simulink model "detumbling"  (R2020a)
settings: Solver=VariableStepAuto  StartTime=0.0  StopTime=3000  RelTol=1e-3
values from neighbouring files (symbols this model uses):
  a = (6371+h)*1e3    (= 6871000)    [AMM_main.m]    (also in Data.m)
  A_RW = sqrt([prop1;prop2;prop3]/(prop1+prop2+prop3))    [AMM_main.m]    (also in Data.m)
  A_t = [Ax;Ay;Az;Ax;Ay;Az;A_sp;A_sp;A_sp;A_sp;]    [AMM_main.m]    (also in Data.m)
  alpha = 0.005    [AMM_main.m]    (also in Data.m = 0.5)
  cd = 2.2    [AMM_main.m]    (also in Data.m)
  init_DCM = DCM0_track    [AMM_main.m]    (also in Data.m = [0.097540404999410   0.957506835434298   0.970592781760616)
  init_orb = orb0_track    [AMM_main.m]    (also in Data.m = [e0,i0,O0,o0,th0])
  init_tumbl = w0_track    [AMM_main.m]    (also in Data.m = 10*pi/180*dir)
  Ir = 1e-7    (= 1e-07)    [AMM_main.m]    (also in Data.m)
  Iz = 2e-7    (= 2e-07)    [AMM_main.m]    (also in Data.m)
  J = [Jx;Jy;Jz]    [AMM_main.m]    (also in Data.m)
  k_mt = 1e10    (= 10000000000)    [AMM_main.m]    (also in Data.m = 1000000)
  k_RW = .1    (= 0.1)    [AMM_main.m]    (also in Data.m = 1)
  max_mx = 1.19    [AMM_main.m]    (also in Data.m)
  max_my = 1.19    [AMM_main.m]    (also in Data.m)
  max_mz = 1.19    [AMM_main.m]    (also in Data.m)
  n = sqrt( mu / a^3 )    [AMM_main.m]    (also in Data.m)
  rho = [rho_sMB;rho_dMB;rho_sSP;rho_dSP]    [AMM_main.m]    (also in Data.m)
  rho_air = 4.39e-16 * 1e6/1e3    (= 4.39e-13)    [AMM_main.m]    (also in Data.m)
  RW_Ir = 3.4e-4    (= 0.00034)    [AMM_main.m]    (also in Data.m)
  RW_max_momentum = 400e-3    (= 0.4)    [AMM_main.m]    (also in Data.m)
  RW_max_torque = 100e-3    (= 0.1)    [AMM_main.m]    (also in Data.m)
  wr = 100*pi/180    (= 1.74532925199)    [AMM_main.m]    (also in Data.m)
  ww_earth = 2*pi/(24*3600)*[0;0;1]    [AMM_main.m]    (also in Data.m)
libraries: simulink x6, vrlib x3
settings Model: Creator=alejandrodemiguelmendiola  LastModifiedBy=alejandrodemiguelmendiola

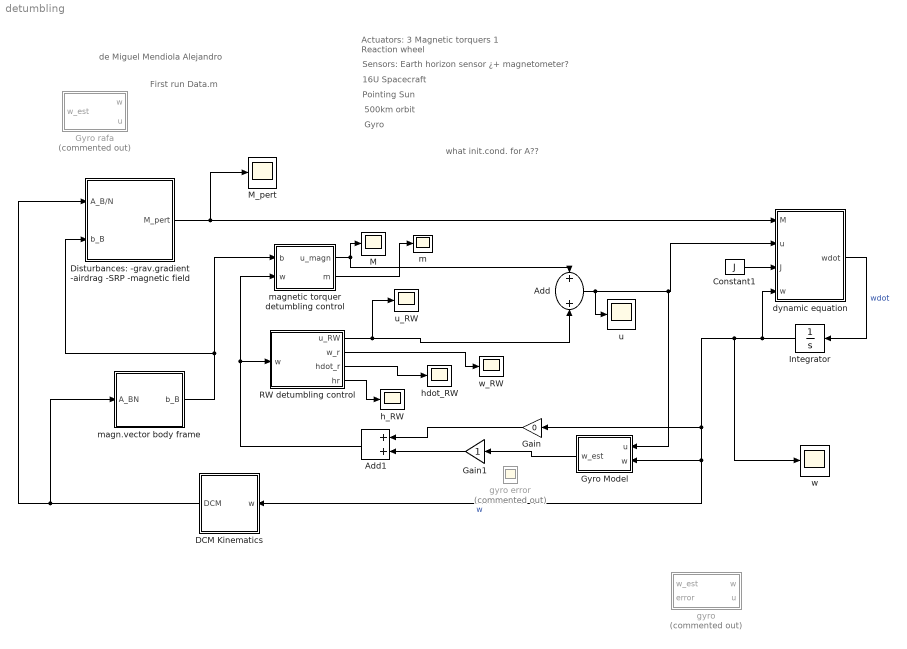
== system detumbling ==
  note: what init.cond. for A??
  note: First run Data.m
  note: Gyro
  note: 500km orbit
  note: Pointing Sun
  note: 16U Spacecraft
  note: Sensors: Earth horizon sensor ¿+ magnetometer?
  note: Actuators: 3 Magnetic torquers
      | 		  1 Reaction wheel
  note: de Miguel Mendiola Alejandro
  Add : Sum
  Add1 : Sum
  Constant1 : Constant  Value=J
  DCM Kinematics : Subsystem
  Disturbances: -grav.gradient -airdrag -SRP -magnetic field : Subsystem
  Gain : Gain  Gain=0
  Gain1 : Gain
  Gyro Model : Subsystem
  Gyro rafa : Subsystem  Commented=on
  Integrator : Integrator  InitialCondition=init_tumbl
  M : Scope
  M_pert : Scope
  RW detumbling control : Subsystem
  dynamic equation : MATLAB Function  TreatAsAtomicUnit=on
  gyro : Subsystem  Commented=on
  gyro error : Scope  Commented=on
  h_RW : Scope
  hdot_RW : Scope
  m : Scope
  magn.vector body frame : Subsystem
  magnetic torquer detumbling control : Subsystem
  u : Scope
  u_RW : Scope
  w : Scope
  w_RW : Scope
  wires:
  dynamic equation/1(wdot) -> Integrator/1  "wdot"
  Integrator/1 -> Gyro Model/2(w), DCM Kinematics/1(w), Gain/1, w/1, dynamic equation/4(w)  "w"
  Disturbances: -grav.gradient -airdrag -SRP -magnetic field/1(M_pert) -> M_pert/1, dynamic equation/1(M)
  magnetic torquer detumbling control/1(u_magn) -> Add/1, M/1
  RW detumbling control/1(u_RW) -> Add/2, u_RW/1
  Add/1 -> u/1, dynamic equation/2(u), Gyro Model/1(u)
  RW detumbling control/2(w_r) -> w_RW/1
  RW detumbling control/3(hdot_r) -> hdot_RW/1
  Constant1/1 -> dynamic equation/3(J)
  DCM Kinematics/1(DCM) -> Disturbances: -grav.gradient -airdrag -SRP -magnetic field/1(A_B/N), magn.vector body frame/1(A_BN)
  RW detumbling control/4(hr) -> h_RW/1
  Add1/1 -> magnetic torquer detumbling control/2(w), RW detumbling control/1(w)
  Gain1/1 -> Add1/2
  Gyro Model/1(w_est) -> Gain1/1
  Gain/1 -> Add1/1
  magnetic torquer detumbling control/2(m) -> m/1
  magn.vector body frame/1(b_B) -> Disturbances: -grav.gradient -airdrag -SRP -magnetic field/2(b_B), magnetic torquer detumbling control/1(b)

== system detumbling/DCM Kinematics ==
  w : Inport
  Integrator : Integrator  InitialCondition=init_DCM
  Iterative Orthonormalization : Subsystem
  Product1 : Product  Multiplication=Matrix(*)
  Unary Minus : UnaryMinus
  hat : MATLAB Function  TreatAsAtomicUnit=on
  DCM : Outport
  wires:
  Unary Minus/1 -> Integrator/1  "Adot"
  hat/1(w_hat) -> Product1/1
  Product1/1 -> Unary Minus/1
  w/1 -> hat/1(w)
  Iterative Orthonormalization/1(A_Ortho) -> Product1/2, DCM/1  "A_ortho"
  Integrator/1 -> Iterative Orthonormalization/1(A)  "A"

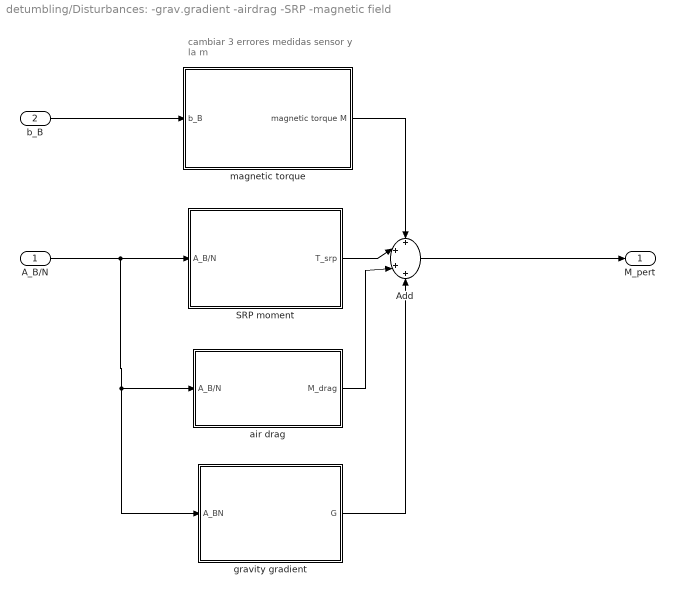
== system detumbling/Disturbances: -grav.gradient -airdrag -SRP -magnetic field ==
  note: cambiar 3 errores medidas sensor
      | y la m
  A_B/N : Inport
  b_B : Inport  Port=2
  Add : Sum  Inputs=++++
  SRP moment : Subsystem
  air drag : Subsystem
  gravity gradient : Subsystem
  magnetic torque : Subsystem
  M_pert : Outport
  wires:
  magnetic torque/1(magnetic torque M) -> Add/1
  A_B/N/1 -> gravity gradient/1(A_BN), air drag/1(A_B/N), SRP moment/1(A_B/N)
  SRP moment/1(T_srp) -> Add/2
  gravity gradient/1(G) -> Add/4
  Add/1 -> M_pert/1
  air drag/1(M_drag) -> Add/3
  b_B/1 -> magnetic torque/1(b_B)

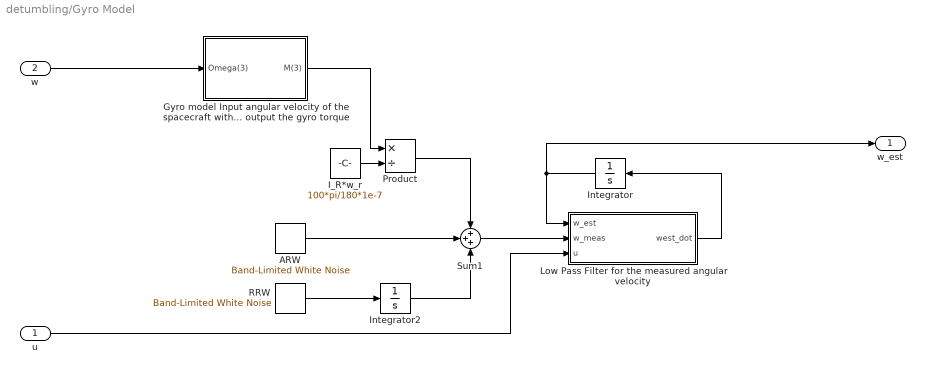
== system detumbling/Gyro Model ==
  u : Inport
  w : Inport  Port=2
  ARW : simulink/Sources/Band-Limited White Noise  Cov=1.9039e-09  Ts=0.0038168  seed=[23341]
  Gyro model Input angular velocity of the spacecraft with output the gyro torque : Subsystem
  I_R*w_r : Constant  Value=100*pi/180*1e-7
  Integrator : Integrator  InitialCondition=[-0.011581;-0.10734;0.13713 ]
  Integrator2 : Integrator  InitialCondition=pi/180/3600*[1,1,1]'
  Low Pass Filter for the measured angular velocity : MATLAB Function  TreatAsAtomicUnit=on
  Product : Product  Inputs=*/
  RRW : simulink/Sources/Band-Limited White Noise  Cov=5.5423e-10  Ts=0.0038168  seed=[23341]
  Sum1 : Sum  Inputs=+++
  w_est : Outport
  wires:
  Gyro model Input angular velocity of the spacecraft with output the gyro torque/1(M(3)) -> Product/1
  Low Pass Filter for the measured angular velocity/1(west_dot) -> Integrator/1
  I_R*w_r/1 -> Product/2
  Integrator/1 -> w_est/1, Low Pass Filter for the measured angular velocity/1(w_est)
  Sum1/1 -> Low Pass Filter for the measured angular velocity/2(w_meas)
  w/1 -> Gyro model Input angular velocity of the spacecraft with output the gyro torque/1(Omega(3))
  u/1 -> Low Pass Filter for the measured angular velocity/3(u)
  Integrator2/1 -> Sum1/3
  Product/1 -> Sum1/1
  RRW/1 -> Integrator2/1
  ARW/1 -> Sum1/2

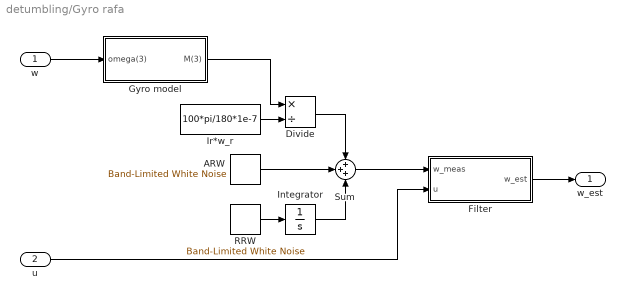
== system detumbling/Gyro rafa ==
  w : Inport
  u : Inport  Port=2
  ARW : simulink/Sources/Band-Limited White Noise  Cov=1.9039e-09  Ts=0.0038168  seed=[23341]
  Divide : Product  Inputs=*/
  Filter : Subsystem
  Gyro model : Subsystem
  Integrator : Integrator  InitialCondition=pi/180/3600*[1 1 1]'
  Ir*w_r : Constant  Value=100*pi/180*1e-7
  RRW : simulink/Sources/Band-Limited White Noise  Cov=5.5423e-10  Ts=0.0038168  seed=[23341]
  Sum : Sum  Inputs=+++
  w_est : Outport
  wires:
  w/1 -> Gyro model/1(omega(3))
  Divide/1 -> Sum/1
  Sum/1 -> Filter/1(w_meas)
  Ir*w_r/1 -> Divide/2
  Gyro model/1(M(3)) -> Divide/1
  u/1 -> Filter/2(u)
  Filter/1(w_est) -> w_est/1
  ARW/1 -> Sum/2
  RRW/1 -> Integrator/1
  Integrator/1 -> Sum/3

== system detumbling/RW detumbling control ==
  w : Inport
  Constant : Constant  Value=k_RW
  detumblingl control of 1 RW : Subsystem
  u_RW : Outport
  w_r : Outport  Port=2
  hdot_r : Outport  Port=3
  hr : Outport  Port=4
  wires:
  w/1 -> detumblingl control of 1 RW/1(w)
  detumblingl control of 1 RW/2(w_r) -> w_r/1
  detumblingl control of 1 RW/1(u_c) -> u_RW/1
  detumblingl control of 1 RW/4(hr) -> hr/1
  detumblingl control of 1 RW/3(hdot_r) -> hdot_r/1
  Constant/1 -> detumblingl control of 1 RW/2(k)

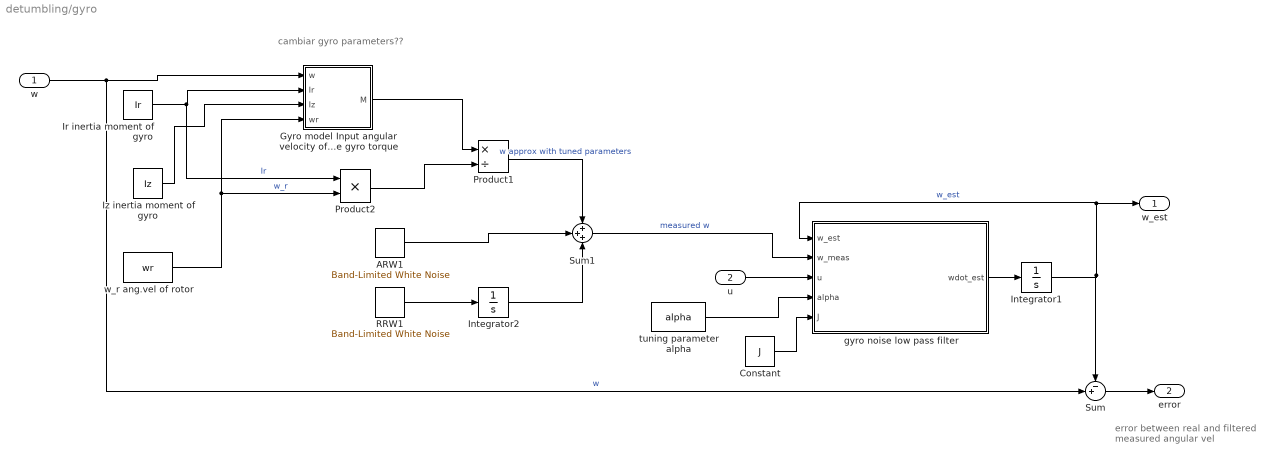
== system detumbling/gyro ==
  note: cambiar gyro parameters??
  note: error between real
      | and filtered measured angular vel
  w : Inport
  u : Inport  Port=2
  ARW1 : simulink/Sources/Band-Limited White Noise  Cov=1.9039e-09  Ts=0.0038168  seed=[23341]
  Constant : Constant  Value=J
  Gyro model Input angular velocity of the spacecraft with output the gyro torque : Subsystem
  Integrator1 : Integrator  InitialCondition=init_tumbl
  Integrator2 : Integrator  InitialCondition=pi/180/3600*[1,1,1]'
  Ir inertia moment of gyro : Constant  Value=Ir
  Iz inertia moment of gyro : Constant  Value=Iz
  Product1 : Product  Inputs=*/
  Product2 : Product  Inputs=**
  RRW1 : simulink/Sources/Band-Limited White Noise  Cov=5.5423e-10  Ts=0.0038168  seed=[23341]
  Sum : Sum  Inputs=-+|
  Sum1 : Sum  Inputs=+++
  gyro noise low pass filter : MATLAB Function  TreatAsAtomicUnit=on
  tuning parameter alpha : Constant  Value=alpha
  w_r ang.vel of rotor : Constant  Value=wr
  w_est : Outport
  error : Outport  Port=2
  wires:
  gyro noise low pass filter/1(wdot_est) -> Integrator1/1
  u/1 -> gyro noise low pass filter/3(u)
  tuning parameter alpha/1 -> gyro noise low pass filter/4(alpha)
  Sum/1 -> error/1
  Product2/1 -> Product1/2
  w/1 -> Gyro model Input angular velocity of the spacecraft with output the gyro torque/1(w), Sum/2  "w"
  Product1/1 -> Sum1/1  "w approx with tuned parameters"
  Integrator1/1 -> Sum/1, w_est/1, gyro noise low pass filter/1(w_est)  "w_est"
  Ir inertia moment of gyro/1 -> Product2/1, Gyro model Input angular velocity of the spacecraft with output the gyro torque/2(Ir)  "Ir"
  w_r ang.vel of rotor/1 -> Product2/2, Gyro model Input angular velocity of the spacecraft with output the gyro torque/4(wr)  "w_r"
  Iz inertia moment of gyro/1 -> Gyro model Input angular velocity of the spacecraft with output the gyro torque/3(Iz)
  Sum1/1 -> gyro noise low pass filter/2(w_meas)  "measured w"
  Gyro model Input angular velocity of the spacecraft with output the gyro torque/1(M) -> Product1/1
  Constant/1 -> gyro noise low pass filter/5(J)
  ARW1/1 -> Sum1/2
  RRW1/1 -> Integrator2/1
  Integrator2/1 -> Sum1/3

== system detumbling/magn.vector body frame ==
  A_BN : Inport
  Clock : Clock
  Constant : Constant  Value=a
  Magnetic model : MATLAB Function  TreatAsAtomicUnit=on
  magn.vector body axis : Subsystem
  s/c position for a given orbit : Subsystem
  b_B : Outport
  wires:
  A_BN/1 -> magn.vector body axis/1(A_BN)
  magn.vector body axis/1(b_B_err) -> b_B/1  "b_B"
  Magnetic model/1(b_N) -> magn.vector body axis/2(b_N)  "b_N"
  s/c position for a given orbit/1(r_N) -> Magnetic model/1(r_N)  "r_N"
  Constant/1 -> s/c position for a given orbit/1(a)
  Clock/1 -> Magnetic model/2(t)

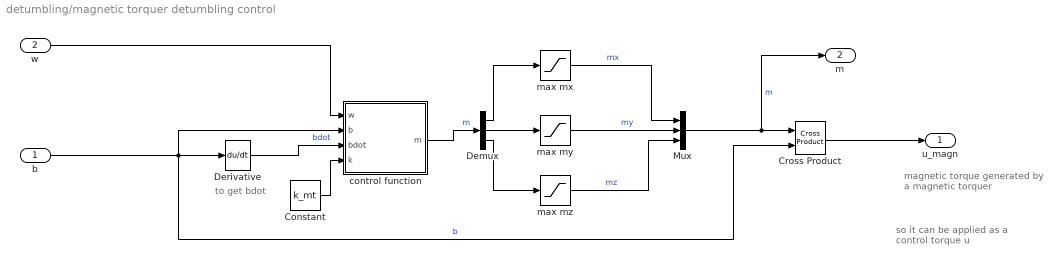
== system detumbling/magnetic torquer detumbling control ==
  note: to get bdot
  note: so it can be applied
      | as a control torque u
  note: magnetic torque
      | generated by a
      | magnetic torquer
  b : Inport
  w : Inport  Port=2
  Constant : Constant  Value=k_mt
  Cross Product : vrlib/Utilities/Cross Product
  Demux : Demux  Outputs=3
  Derivative : Derivative
  Mux : Mux  Inputs=3
  control function : MATLAB Function  TreatAsAtomicUnit=on
  max mx : Saturate  UpperLimit=max_mx  LowerLimit=-max_mx  ZeroCross=off
  max my : Saturate  UpperLimit=max_my  LowerLimit=-max_my  ZeroCross=off
  max mz : Saturate  UpperLimit=max_mz  LowerLimit=-max_mz  ZeroCross=off
  u_magn : Outport
  m : Outport  Port=2
  wires:
  w/1 -> control function/1(w)
  control function/1(m) -> Demux/1  "m"
  b/1 -> control function/2(b), Cross Product/2, Derivative/1  "b"
  Mux/1 -> m/1, Cross Product/1  "m"
  Cross Product/1 -> u_magn/1
  max mx/1 -> Mux/1  "mx"
  max my/1 -> Mux/2  "my"
  max mz/1 -> Mux/3  "mz"
  Demux/1 -> max mx/1
  Demux/2 -> max my/1
  Demux/3 -> max mz/1
  Derivative/1 -> control function/3(bdot)  "bdot"
  Constant/1 -> control function/4(k)

== system detumbling/DCM Kinematics/Iterative Orthonormalization ==
  note: Uncomment if needed
      | With 2 blocks working:
      | Error ~1e-16 up to t=1e6
      | Error ~1e-14 up to t=1e7
  A : Inport
  Ortho DCM : Subsystem
  Ortho DCM1 : Subsystem
  Ortho DCM2 : Subsystem  Commented=through
  Ortho DCM3 : Subsystem  Commented=through
  Ortho DCM4 : Subsystem  Commented=through
  A_Ortho : Outport
  wires:
  Ortho DCM1/1(A_ortho) -> Ortho DCM2/1(A)
  Ortho DCM/1(A_ortho) -> Ortho DCM1/1(A)
  Ortho DCM3/1(A_ortho) -> Ortho DCM4/1(A)
  Ortho DCM2/1(A_ortho) -> Ortho DCM3/1(A)
  A/1 -> Ortho DCM/1(A)
  Ortho DCM4/1(A_ortho) -> A_Ortho/1

== system detumbling/Disturbances: -grav.gradient -airdrag -SRP -magnetic field/SRP moment ==
  A_B/N : Inport
  Area : Constant  Value=A_t
  SRP disturbance torque : MATLAB Function  TreatAsAtomicUnit=on
  Sun direction wrt s/c body frame : Subsystem
  optical properties : Constant  Value=rho
  T_srp : Outport
  wires:
  A_B/N/1 -> Sun direction wrt s/c body frame/1(A_B/N)
  SRP disturbance torque/1(T_srp) -> T_srp/1
  Sun direction wrt s/c body frame/1(S^_B) -> SRP disturbance torque/1(S_B)
  Area/1 -> SRP disturbance torque/2(A)
  optical properties/1 -> SRP disturbance torque/3(rho)

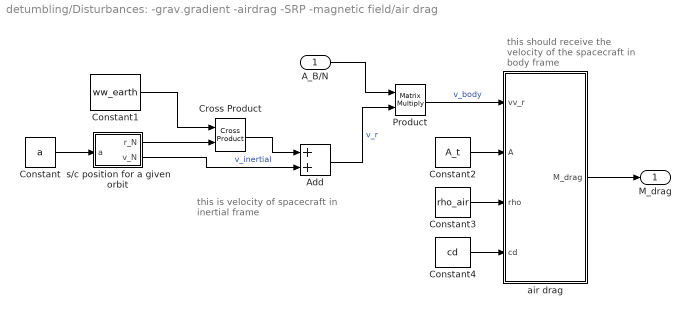
== system detumbling/Disturbances: -grav.gradient -airdrag -SRP -magnetic field/air drag ==
  note: this is velocity
      | of spacecraft in
      | inertial frame
  note: this should receive the
      | velocity of the spacecraft
      | in body frame
  A_B/N : Inport
  Add : Sum
  Constant : Constant  Value=a
  Constant1 : Constant  Value=ww_earth
  Constant2 : Constant  Value=A_t
  Constant3 : Constant  Value=rho_air
  Constant4 : Constant  Value=cd
  Cross Product : vrlib/Utilities/Cross Product
  Product : Product  Multiplication=Matrix(*)
  air drag : MATLAB Function  TreatAsAtomicUnit=on
  s/c position for a given orbit : Subsystem
  M_drag : Outport
  wires:
  air drag/1(M_drag) -> M_drag/1
  A_B/N/1 -> Product/1
  Product/1 -> air drag/1(vv_r)  "v_body"
  Constant/1 -> s/c position for a given orbit/1(a)
  s/c position for a given orbit/1(r_N) -> Cross Product/2
  Constant1/1 -> Cross Product/1
  Cross Product/1 -> Add/1
  s/c position for a given orbit/2(v_N) -> Add/2  "v_inertial"
  Add/1 -> Product/2  "v_r"
  Constant2/1 -> air drag/2(A)
  Constant4/1 -> air drag/4(cd)
  Constant3/1 -> air drag/3(rho)

== system detumbling/Disturbances: -grav.gradient -airdrag -SRP -magnetic field/gravity gradient ==
  A_BN : Inport
  A_N/L : Subsystem
  Product : Product  Multiplication=Matrix(*)
  gravity gradient : MATLAB Function  TreatAsAtomicUnit=on
  mean motion : Constant  Value=n
  moment of inertia : Constant  Value=J
  G : Outport
  wires:
  gravity gradient/1(G) -> G/1
  A_N/L/1(A_N/L) -> Product/2
  A_BN/1 -> Product/1
  Product/1 -> gravity gradient/1(A_BL)
  moment of inertia/1 -> gravity gradient/2(J)
  mean motion/1 -> gravity gradient/3(n)

== system detumbling/Disturbances: -grav.gradient -airdrag -SRP -magnetic field/magnetic torque ==
  b_B : Inport
  Cross Product : vrlib/Utilities/Cross Product
  m (worst case scenario) : Constant  Value=[0.1;0.1;0.1]
  m (from labs) : Constant  Commented=on  Value=[0.01;0.05;0.01]
  magnetic torque M : Outport
  wires:
  b_B/1 -> Cross Product/2  "b_B"
  m (worst case scenario)/1 -> Cross Product/1
  Cross Product/1 -> magnetic torque M/1  "M"

== system detumbling/Gyro Model/Gyro model Input angular velocity of the spacecraft with output the gyro torque ==
  Omega(3) : Inport
  Integrator2 : Integrator  InitialCondition=[0 0 0 0 0 0]'
  MATLAB Function1 : MATLAB Function  TreatAsAtomicUnit=on
  M(3) : Outport
  wires:
  Integrator2/1 -> MATLAB Function1/1(x)
  MATLAB Function1/1(x_dot) -> Integrator2/1
  Omega(3)/1 -> MATLAB Function1/2(om)
  MATLAB Function1/2(M) -> M(3)/1

== system detumbling/Gyro rafa/Filter ==
  w_meas : Inport
  u : Inport  Port=2
  Integrator : Integrator  InitialCondition=[-0.0157; -0.1329; 0.1121]
  MATLAB Function : MATLAB Function  TreatAsAtomicUnit=on
  w_est : Outport
  wires:
  MATLAB Function/1(west_dot) -> Integrator/1
  Integrator/1 -> w_est/1, MATLAB Function/3(w_est)
  w_meas/1 -> MATLAB Function/1(w_meas)
  u/1 -> MATLAB Function/2(u)

== system detumbling/Gyro rafa/Gyro model ==
  omega(3) : Inport
  Integrator : Integrator  InitialCondition=zeros(6,1)
  MATLAB Function : MATLAB Function  TreatAsAtomicUnit=on
  Scope : Scope
  Scope1 : Scope
  M(3) : Outport
  wires:
  MATLAB Function/2(M) -> M(3)/1
  omega(3)/1 -> MATLAB Function/2(w)
  MATLAB Function/1(x_dot) -> Scope/1, Integrator/1
  Integrator/1 -> Scope1/1, MATLAB Function/1(x)

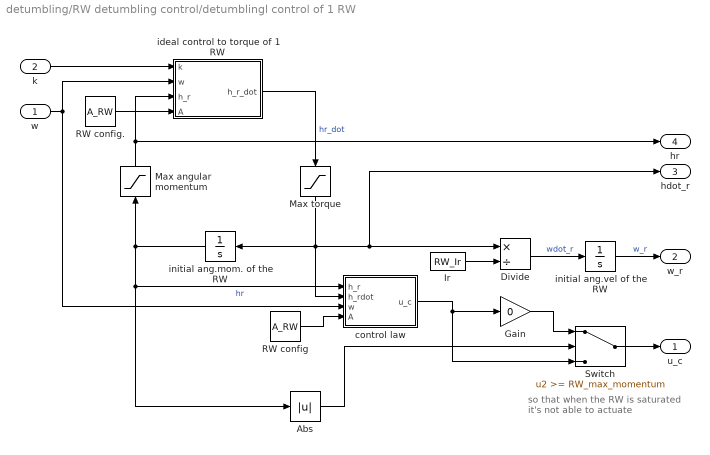
== system detumbling/RW detumbling control/detumblingl control of 1 RW ==
  note: so that when the RW is saturated
      | it's not able to actuate
  w : Inport
  k : Inport  Port=2
  Abs : Abs
  Divide : Product  Inputs=*/
  Gain : Gain  Gain=0
  Ir : Constant  Value=RW_Ir
  Max angular momentum : Saturate  UpperLimit=RW_max_momentum  LowerLimit=-RW_max_momentum
  Max torque : Saturate  UpperLimit=RW_max_torque  LowerLimit=-RW_max_torque
  RW config : Constant  Value=A_RW
  RW config. : Constant  Value=A_RW
  Switch : Switch  Threshold=RW_max_momentum
  control law : MATLAB Function  TreatAsAtomicUnit=on
  ideal control to torque of 1 RW : MATLAB Function  TreatAsAtomicUnit=on
  "initial ang.mom. of the RW " : Integrator
  initial ang.vel of the RW : Integrator
  u_c : Outport
  w_r : Outport  Port=2
  hdot_r : Outport  Port=3
  hr : Outport  Port=4
  wires:
  k/1 -> ideal control to torque of 1 RW/1(k)
  w/1 -> ideal control to torque of 1 RW/2(w), control law/3(w)
  ideal control to torque of 1 RW/1(h_r_dot) -> Max torque/1  "hr_dot"
  "initial ang.mom. of the RW "/1 -> Max angular momentum/1, Abs/1, control law/1(h_r)  "hr"
  Max torque/1 -> "initial ang.mom. of the RW "/1, control law/2(h_rdot), hdot_r/1, Divide/1
  Max angular momentum/1 -> hr/1, ideal control to torque of 1 RW/3(h_r)
  Ir/1 -> Divide/2
  Divide/1 -> initial ang.vel of the RW/1  "wdot_r"
  initial ang.vel of the RW/1 -> w_r/1  "w_r"
  RW config/1 -> control law/4(A)
  RW config./1 -> ideal control to torque of 1 RW/4(A)
  Abs/1 -> Switch/2
  Switch/1 -> u_c/1
  control law/1(u_c) -> Gain/1, Switch/3
  Gain/1 -> Switch/1

== system detumbling/gyro/Gyro model Input angular velocity of the spacecraft with output the gyro torque ==
  w : Inport
  Ir : Inport  Port=2
  Iz : Inport  Port=3
  wr : Inport  Port=4
  Integrator2 : Integrator  InitialCondition=[0;0;0;0;0;0]
  MATLAB Function1 : MATLAB Function  TreatAsAtomicUnit=on
  M : Outport
  wires:
  Integrator2/1 -> MATLAB Function1/4(x)
  MATLAB Function1/1(x_dot) -> Integrator2/1
  w/1 -> MATLAB Function1/5(w)
  MATLAB Function1/2(M) -> M/1
  Ir/1 -> MATLAB Function1/1(Ir)
  Iz/1 -> MATLAB Function1/2(Iz)
  wr/1 -> MATLAB Function1/3(w_r)

== system detumbling/magn.vector body frame/magn.vector body axis ==
  A_BN : Inport
  b_N : Inport  Port=2
  Product : Product  Multiplication=Matrix(*)
  b_B_err : Outport
  wires:
  A_BN/1 -> Product/1
  b_N/1 -> Product/2
  Product/1 -> b_B_err/1

== system detumbling/magn.vector body frame/s//c position for a given orbit ==
  a : Inport
  Earth's position : MATLAB Function  TreatAsAtomicUnit=on
  orb_elements dynamics : Subsystem
  r_N : Outport
  v_N : Outport  Port=2
  wires:
  Earth's position/1(r_N) -> r_N/1  "r_N"
  orb_elements dynamics/1(orb_elements) -> Earth's position/2(orb_elements)
  a/1 -> orb_elements dynamics/1(a), Earth's position/1(a)  "a"
  Earth's position/2(v_N) -> v_N/1

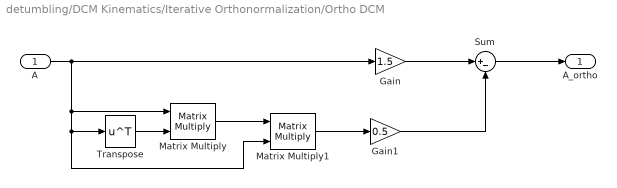
== system detumbling/DCM Kinematics/Iterative Orthonormalization/Ortho DCM ==
  A : Inport
  Gain : Gain  Gain=1.5
  Gain1 : Gain  Gain=0.5
  Matrix Multiply : Product  Multiplication=Matrix(*)
  Matrix Multiply1 : Product  Multiplication=Matrix(*)
  Sum : Sum  Inputs=|+-
  Transpose : Math  Operator=transpose  SaturateOnIntegerOverflow=on
  A_ortho : Outport
  wires:
  Sum/1 -> A_ortho/1
  Gain/1 -> Sum/1
  A/1 -> Matrix Multiply1/2, Transpose/1, Matrix Multiply/1, Gain/1
  Gain1/1 -> Sum/2
  Transpose/1 -> Matrix Multiply/2
  Matrix Multiply/1 -> Matrix Multiply1/1
  Matrix Multiply1/1 -> Gain1/1

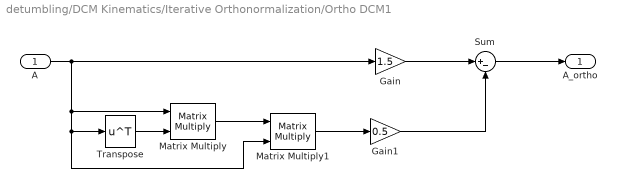
== system detumbling/DCM Kinematics/Iterative Orthonormalization/Ortho DCM1 ==
  A : Inport
  Gain : Gain  Gain=1.5
  Gain1 : Gain  Gain=0.5
  Matrix Multiply : Product  Multiplication=Matrix(*)
  Matrix Multiply1 : Product  Multiplication=Matrix(*)
  Sum : Sum  Inputs=|+-
  Transpose : Math  Operator=transpose  SaturateOnIntegerOverflow=on
  A_ortho : Outport
  wires:
  Sum/1 -> A_ortho/1
  Gain/1 -> Sum/1
  A/1 -> Matrix Multiply1/2, Transpose/1, Matrix Multiply/1, Gain/1
  Gain1/1 -> Sum/2
  Transpose/1 -> Matrix Multiply/2
  Matrix Multiply/1 -> Matrix Multiply1/1
  Matrix Multiply1/1 -> Gain1/1

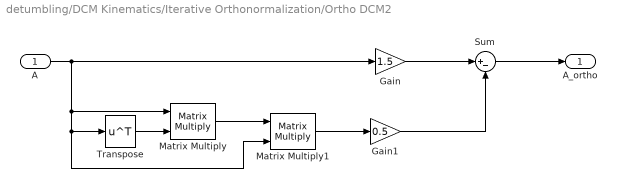
== system detumbling/DCM Kinematics/Iterative Orthonormalization/Ortho DCM2 ==
  A : Inport
  Gain : Gain  Gain=1.5
  Gain1 : Gain  Gain=0.5
  Matrix Multiply : Product  Multiplication=Matrix(*)
  Matrix Multiply1 : Product  Multiplication=Matrix(*)
  Sum : Sum  Inputs=|+-
  Transpose : Math  Operator=transpose  SaturateOnIntegerOverflow=on
  A_ortho : Outport
  wires:
  Sum/1 -> A_ortho/1
  Gain/1 -> Sum/1
  A/1 -> Matrix Multiply1/2, Transpose/1, Matrix Multiply/1, Gain/1
  Gain1/1 -> Sum/2
  Transpose/1 -> Matrix Multiply/2
  Matrix Multiply/1 -> Matrix Multiply1/1
  Matrix Multiply1/1 -> Gain1/1

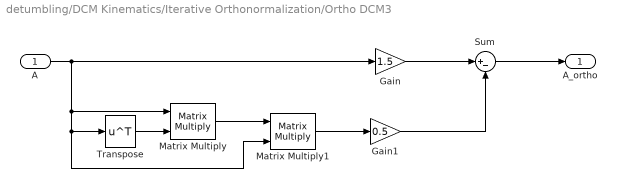
== system detumbling/DCM Kinematics/Iterative Orthonormalization/Ortho DCM3 ==
  A : Inport
  Gain : Gain  Gain=1.5
  Gain1 : Gain  Gain=0.5
  Matrix Multiply : Product  Multiplication=Matrix(*)
  Matrix Multiply1 : Product  Multiplication=Matrix(*)
  Sum : Sum  Inputs=|+-
  Transpose : Math  Operator=transpose  SaturateOnIntegerOverflow=on
  A_ortho : Outport
  wires:
  Sum/1 -> A_ortho/1
  Gain/1 -> Sum/1
  A/1 -> Matrix Multiply1/2, Transpose/1, Matrix Multiply/1, Gain/1
  Gain1/1 -> Sum/2
  Transpose/1 -> Matrix Multiply/2
  Matrix Multiply/1 -> Matrix Multiply1/1
  Matrix Multiply1/1 -> Gain1/1

== system detumbling/DCM Kinematics/Iterative Orthonormalization/Ortho DCM4 ==
  A : Inport
  Gain : Gain  Gain=1.5
  Gain1 : Gain  Gain=0.5
  Matrix Multiply : Product  Multiplication=Matrix(*)
  Matrix Multiply1 : Product  Multiplication=Matrix(*)
  Sum : Sum  Inputs=|+-
  Transpose : Math  Operator=transpose  SaturateOnIntegerOverflow=on
  A_ortho : Outport
  wires:
  Sum/1 -> A_ortho/1
  Gain/1 -> Sum/1
  A/1 -> Matrix Multiply1/2, Transpose/1, Matrix Multiply/1, Gain/1
  Gain1/1 -> Sum/2
  Transpose/1 -> Matrix Multiply/2
  Matrix Multiply/1 -> Matrix Multiply1/1
  Matrix Multiply1/1 -> Gain1/1

== system detumbling/Disturbances: -grav.gradient -airdrag -SRP -magnetic field/SRP moment/Sun direction wrt s//c body frame ==
  A_B/N : Inport
  Clock : Clock
  Product3 : Product  Multiplication=Matrix(*)
  Sun's direction : MATLAB Function  TreatAsAtomicUnit=on
  S^_B : Outport
  wires:
  Product3/1 -> S^_B/1
  A_B/N/1 -> Product3/1
  Clock/1 -> Sun's direction/1(t)
  Sun's direction/1(S_N) -> Product3/2  "S^_N"

== system detumbling/Disturbances: -grav.gradient -airdrag -SRP -magnetic field/air drag/s//c position for a given orbit ==
  a : Inport
  Earth's position : MATLAB Function  TreatAsAtomicUnit=on
  orb_elements dynamics : Subsystem
  r_N : Outport
  v_N : Outport  Port=2
  wires:
  Earth's position/1(r_N) -> r_N/1  "r_N"
  orb_elements dynamics/1(orb_elements) -> Earth's position/2(orb_elements)
  a/1 -> orb_elements dynamics/1(a), Earth's position/1(a)  "a"
  Earth's position/2(v_N) -> v_N/1

== system detumbling/Disturbances: -grav.gradient -airdrag -SRP -magnetic field/gravity gradient/A_N//L ==
  Clock : Clock
  MATLAB Function1 : MATLAB Function  TreatAsAtomicUnit=on
  Transpose : Math  Operator=transpose  SaturateOnIntegerOverflow=on
  mean motion : Constant  Value=n
  A_N/L : Outport
  wires:
  Transpose/1 -> A_N/L/1  "A_N/L"
  Clock/1 -> MATLAB Function1/1(t)
  MATLAB Function1/1(A_LN) -> Transpose/1  "A_LN"
  mean motion/1 -> MATLAB Function1/2(n)

== system detumbling/magn.vector body frame/s//c position for a given orbit/orb_elements dynamics ==
  a : Inport
  Integrator : Integrator  InitialCondition=init_orb
  sat motion : MATLAB Function  TreatAsAtomicUnit=on
  orb_elements : Outport
  wires:
  Integrator/1 -> sat motion/2(orb_elements), orb_elements/1  "orb_elements"
  sat motion/1(orb_elements_dot) -> Integrator/1
  a/1 -> sat motion/1(a)

== system detumbling/Disturbances: -grav.gradient -airdrag -SRP -magnetic field/air drag/s//c position for a given orbit/orb_elements dynamics ==
  a : Inport
  Integrator : Integrator  InitialCondition=init_orb
  sat motion : MATLAB Function  TreatAsAtomicUnit=on
  orb_elements : Outport
  wires:
  Integrator/1 -> sat motion/2(orb_elements), orb_elements/1  "orb_elements"
  sat motion/1(orb_elements_dot) -> Integrator/1
  a/1 -> sat motion/1(a)

== matlab function detumbling/Gyro Model/Gyro model Input angular velocity of the spacecraft with output the gyro torque/MATLAB Function1 ==
  data: x input; om input; x_dot output; M output
function [x_dot,M]  = Gyro(x,om)
%gyro inertia parameters 
Ir = 1e-7; 
Iz = 2e-7;
%tuning parameter for visco-elastic reaction torque
k_gyro=10;
%tuning law for c for fastest convergence
c_gyro = 2*sqrt(k_gyro*Iz); 
om_x = om(1); 
om_y = om(2); 
om_z = om(3); 
%angular velocity of gyro wheel
om_r = 100*pi/180;

% defining the theta_i and \dot theta_i 
x_dot = zeros(6,1); 

th_x = x(1); 
th_y = x(2); 
th_z = x(3);
va_x = x(4);
va_y = x(5); 
va_z = x(6); 
%3 gyro dynamics expressed as 1st order differential equation
x_dot(1) = va_x;
x_dot(2) = va_y; 
x_dot(3) = va_z;
x_dot(4) = -(c_gyro/Iz)*va_x-(k_gyro/Iz)*th_x-(Ir/Iz)*om_r*om_x;
x_dot(5) = -(c_gyro/Iz)*va_y-(k_gyro/Iz)*th_y-(Ir/Iz)*om_r*om_y;
x_dot(6) = -(c_gyro/Iz)*va_z-(k_gyro/Iz)*th_z-(Ir/Iz)*om_r*om_z;
%gyro outputs 
x_dot=[x_dot(1) x_dot(2) x_dot(3) x_dot(4) x_dot(5) x_dot(6)]';
%feedback torque applied to the gyros 
M_x = -k_gyro*th_x-c_gyro*va_x;
M_y = -k_gyro*th_y-c_gyro*va_y;
M_z = -k_gyro*th_z-c_gyro*va_z;

M = [M_x M_y M_z]'; 


end

== matlab function detumbling/magnetic torquer detumbling control/control function ==
  data: w input; m output; b input; bdot input; k input
function m = fcn(w,b,bdot,k) %add bdot input if want to implement control '1' or '2'

%DIFFERENT FEEDBACK CONTROLS
type = 1;
switch type
    case 1
%         k = 5e5;
        m = -k*bdot;
    case 2
        m_max = 0.31; %[Am^2] Maximum magnetic dipole moment. In lab slides it says 3.5 but it's too much for a cubesat        
        eps = 1e-6;
        m = zeros(size(bdot));
        for i = 1:3
            if abs(bdot(i))>eps
             m(i) = -m_max*sign(bdot(i)); %control law magnetic torquer on/off
            end
        end
        
    case 3
%         k = 1e5;
        m = -k*cross(b,w); %using the approximation of: bdot = cross(b,w); in real life it has the disadvantage
        %having to know w, so you need a gyro to know it.
end

== matlab function detumbling/gyro/Gyro model Input angular velocity of the spacecraft with output the gyro torque/MATLAB Function1 ==
  data: Ir input; Iz input; w_r input; x input; w input; x_dot output; M output
function [x_dot,M]  = Gyro(Ir,Iz,w_r,x,w)
%DATA
% Ir = 1e-7; %gyro inertia parameters 
% Iz = 2e-7;
% w_r = 100*pi/180; %angular velocity of gyro wheel
k_gyro=10; %tuning parameter for visco-elastic reaction torque
c_gyro = 2*sqrt(k_gyro*Iz); 


%tuning law for c for fastest convergence
w_x = w(1); %angular velocity in body frame 
w_y = w(2); 
w_z = w(3); 

% defining the theta_i and \dot theta_i 
x_dot = zeros(6,1); % x will be the state variable
th_x = x(1); %turning angle of the gyro
th_y = x(2); 
th_z = x(3);
va_x = x(4); %angular velocity of the gyro
va_y = x(5); 
va_z = x(6); 

%3 gyro dynamics expressed as 1st order differential equation
x_dot(1) = va_x;
x_dot(2) = va_y; 
x_dot(3) = va_z;
x_dot(4) = -(c_gyro/Iz)*va_x-(k_gyro/Iz)*th_x-(Ir/Iz)*w_r*w_x;
x_dot(5) = -(c_gyro/Iz)*va_y-(k_gyro/Iz)*th_y-(Ir/Iz)*w_r*w_y;
x_dot(6) = -(c_gyro/Iz)*va_z-(k_gyro/Iz)*th_z-(Ir/Iz)*w_r*w_z;


%feedback torque applied to the gyros 
M = zeros(3,1);
M(1) = -k_gyro*th_x-c_gyro*va_x;
M(2) = -k_gyro*th_y-c_gyro*va_y;
M(3) = -k_gyro*th_z-c_gyro*va_z;


end %function

== matlab function detumbling/gyro/gyro noise low pass filter ==
  data: w_est input; w_meas input; u input; wdot_est output; alpha input; J input
function wdot_est = fcn(w_est,w_meas,u,alpha,J)

% J1 = 100.9e-2;
% J2 =  25.1e-2;
% J3 =  91.6e-2;
J1 = J(1);
J2 = J(2);
J3 = J(3);

wdot_est = zeros(size(w_est));

wdot_est(1) =       (J2 - J3)/J1 * w_est(2) * w_est(3) + u(1)/J1 - ...
                alpha*(w_est(1)-w_meas(1))/J1;
wdot_est(2) =       (J3 - J1)/J2 * w_est(1) * w_est(3) + u(2)/J2 - ...
                alpha*(w_est(2)-w_meas(2))/J2;
wdot_est(3) =       (J1 - J2)/J3 * w_est(1) * w_est(2) + u(3)/J3 - ...
                alpha*(w_est(3)-w_meas(3))/J3;

    
end

== matlab function detumbling/Gyro Model/Low Pass Filter for the measured angular velocity ==
  data: w_est input; w_meas input; u input; west_dot output
function west_dot = dynamics(w_est,w_meas,u)

J1 = 0.1054;
J2 = 0.0914;
J3 = 0.0541;

alpha = 0.004;

west_dot = zeros(size(w_est));

west_dot(1) =       (J2 - J3)/J1 * w_est(2) * w_est(3) + u(1)/J1 - ...
                alpha*(w_est(1)-w_meas(1))/J1;
west_dot(2) =       (J3 - J1)/J2 * w_est(1) * w_est(3) + u(2)/J2 - ...
                alpha*(w_est(2)-w_meas(2))/J2;
west_dot(3) =       (J1 - J2)/J3 * w_est(1) * w_est(2) + u(3)/J3 - ...
                alpha*(w_est(3)-w_meas(3))/J3;

== matlab function detumbling/RW detumbling control/detumblingl control of 1 RW/control law ==
  data: h_r input; h_rdot input; w input; u_c output; A input
function u_c = fcn(h_r,h_rdot,w,A)

% A = [1/sqrt(3);1/sqrt(3);1/sqrt(3)]; % one single Reaction wheel equal
% configuration

u_c = zeros(3,1);
u_c = -A*h_rdot-cross(w,A*h_r);

== matlab function detumbling/magn.vector body frame/Magnetic model ==
  data: r_N input; b_N output; t input
function b_N = fcn(r_N,t)
% coefficients
IGRF = '2000';
switch IGRF
    case '1995'
        g0_1 = -29682e-9;
        g1_1 = -1789e-9;
        h1_1 = 5318e-9;
    case '2000'
        g0_1 = -29615e-9;
        g1_1 = -1728e-9;
        h1_1 = 5186e-9;
end


w = 360/(24*3600) * pi/180; %[rad/s] angular rotation speed of Earth
decl = 11.5*pi/180; %[rad]
R = 6371.2e3; %equatorial radius [m]
r = norm(r_N);
rr_unit = r_N/r; %unitary vector

H0 = sqrt(g0_1^2 + g1_1^2 + h1_1^2);
m = [
    sin(decl)*cos(w*t);
    sin(decl)*sin(w*t);
    cos(decl)
    ]; %unit vector along dipole axis

b_N = R^3*H0/r^3*(3*(dot(m,rr_unit))*rr_unit - m); %Earth's MF in the inertial frame

== matlab function detumbling/Disturbances: -grav.gradient -airdrag -SRP -magnetic field/SRP moment/Sun direction wrt s//c body frame/Sun's direction ==
  data: t input; S_N output
function S_N = fcn(t)

%% data
Rs = 149597870700; %[m] but we can substitute it by 1 so we have a unitary vector
Rs = 1;
epsilon = 23.45 * pi/180; %[rad]
T = 365.25*24*3600; %[s]
nsun = 2*pi/T; % [s^-1]

%% 
S_N = Rs * [cos(nsun*t);
            sin(nsun*t)*cos(epsilon);
            sin(nsun*t)*sin(epsilon);];

end

== matlab function detumbling/Gyro rafa/Filter/MATLAB Function ==
  data: w_meas input; u input; w_est input; west_dot output
function west_dot = dynamics(w_meas, u, w_est)

% J1 = 0.0547;
% J2 = 0.0519;
% J3 = 0.0574; % https://issfd.org/ISSFD_2014/ISSFD24_Paper_S1-4_carrara.pdf
J1 = 100.9e-2;
J2 =  25.1e-2;
J3 =  91.6e-2;

alpha = 2;

west_dot = zeros(size(w_est));

west_dot(1) = (J2 - J3)/J1*w_est(2)*w_est(3) + u(1)/J1 - ...
                                           alpha*(w_est(1) - w_meas(1))/J1;
west_dot(2) = (J3 - J1)/J2*w_est(1)*w_est(3) + u(2)/J2 - ...
                                           alpha*(w_est(2) - w_meas(2))/J2;
west_dot(3) = (J1 - J2)/J3*w_est(1)*w_est(2) + u(3)/J3 - ...
                                           alpha*(w_est(3) - w_meas(3))/J3;

== matlab function detumbling/Gyro rafa/Gyro model/MATLAB Function ==
  data: x_dot output; x input; w input; M output
function [x_dot, M]= gyro(x, w)

Ir = 1e-7;
Iz = 2e-7;

k = 10;
c = 2*sqrt(k*Iz);

w_x = w(1);
w_y = w(2);
w_z = w(3);
w_r = 100*pi/180;

t_x = x(1); 
t_y = x(2); 
t_z = x(3);
tdot_x = x(4);
tdot_y = x(5); 
tdot_z = x(6); 

x_dot = zeros(6,1);

x_dot(1) = tdot_x;
x_dot(2) = tdot_y; 
x_dot(3) = tdot_z;
x_dot(4) = -(c/Iz)*tdot_x - (k/Iz)*t_x - (Ir/Iz)*w_r*w_x;
x_dot(5) = -(c/Iz)*tdot_y - (k/Iz)*t_y - (Ir/Iz)*w_r*w_y;
x_dot(6) = -(c/Iz)*tdot_z - (k/Iz)*t_z - (Ir/Iz)*w_r*w_z;

M_x = -k*t_x - c*tdot_x;
M_y = -k*t_y - c*tdot_y;
M_z = -k*t_z - c*tdot_z;

M = [M_x M_y M_z]';

== matlab function detumbling/Disturbances: -grav.gradient -airdrag -SRP -magnetic field/gravity gradient/A_N//L/MATLAB Function1 ==
  data: t input; A_LN output; n input
function A_LN = fcn(t,n)

% mu = 3.986004418e14;
% n = sqrt( mu / a^3 ); %is this the nº of revolutions per orbit?
A_LN = [cos(n*t) sin(n*t) 0;
    -sin(n*t) cos(n*t) 0;
    0 0 1;
    ];

== matlab function detumbling/RW detumbling control/detumblingl control of 1 RW/ideal control to torque of 1 RW ==
  data: k input; h_r_dot output; w input; h_r input; A input
function h_r_dot = fcn(k,w,h_r,A)

% A = [1/sqrt(3);1/sqrt(3);1/sqrt(3)]; % one single Reaction wheel
% configuration

%detumbling law
u = -k*w;

Apseudo_inv = pinv(A);

h_r_dot = 0;
h_r_dot = -Apseudo_inv*(u+cross(w,A*h_r));

== matlab function detumbling/Disturbances: -grav.gradient -airdrag -SRP -magnetic field/gravity gradient/gravity gradient ==
  data: A_BL input; G output; J input; n input
function G = fcn(A_BL,J,n)

%Data
% mu = 3.986004418e14;
% n  = sqrt(mu/a^3);
% %Moment of inertia of s/c
% Ix = 100.9e-2; %[kg m^2]
% Iy = 25.1e-2;
% Iz = 91.6e-2; 
Ix = J(1);
Iy = J(2);
Iz = J(3);
c = A_BL * [1;0;0];

G = zeros(3,1);
G(1) = 3*n^2 * (Iz - Iy)*c(3)*c(2);
G(2) = 3*n^2 * (Ix - Iz)*c(1)*c(3);
G(3) = 3*n^2 * (Iy - Ix)*c(2)*c(1);

end

== matlab function detumbling/magn.vector body frame/s//c position for a given orbit/Earth's position ==
  data: a input; orb_elements input; r_N output; v_N output
function [r_N,v_N]  = Earth_pos(a,orb_elements)

mu = 3.986004418e14;

e_mod = orb_elements(1);
i     = orb_elements(2);
Omega = orb_elements(3);
omega = orb_elements(4);
theta = orb_elements(5);


h_mod = sqrt(mu*a*(1-e_mod^2));
    
e_unit = rotation_matrix_R3(-Omega) * ...
         rotation_matrix_R1(-i) * ...
         rotation_matrix_R3(-omega) * [1;0;0];
p_unit = rotation_matrix_R3(-Omega) * ...
         rotation_matrix_R1(-i) * ...
         rotation_matrix_R3(-omega) * [0;1;0];
     
r_mod_0 = h_mod^2/mu/(1+e_mod*cos(theta));
r_N       = r_mod_0 * ( cos(theta) * e_unit  +  sin(theta) * p_unit );
v_r     = mu/h_mod * e_mod*sin(theta);
v_theta = mu/h_mod * (1 + e_mod*cos(theta));
v_N       = v_r     * (  cos(theta) * e_unit  +  sin(theta) * p_unit )+ ...
          v_theta * ( -sin(theta) * e_unit  +  cos(theta) * p_unit );
end


function R1 = rotation_matrix_R1(alpha)
%{
rotation_matrix_R1: computes rotation matrix of angle alpha around x axis

INPUT:
	alpha[1]                Angle rotated
                                [rad]

OUTPUT:
    R1 [3x3]                Rotation matrix
                                [(3x3) x -]
%}

R1 = zeros(3);

R1(1,1) = 1;
R1(2,2) =  cos(alpha);
R1(2,3) =  sin(alpha);
R1(3,2) = -sin(alpha);
R1(3,3) =  cos(alpha);
end


function R3 = rotation_matrix_R3(alpha)
%{
rotation_matrix_R3: computes rotation matrix of angle alpha around z axis

INPUT:
	alpha[1]                Angle rotated
                                [rad]

OUTPUT:
    R3 [3x3]                Rotation matrix
                                [(3x3) x -]

%}

R3 = zeros(3);

R3(1,1) =  cos(alpha);
R3(1,2) =  sin(alpha);
R3(2,1) = -sin(alpha);
R3(2,2) =  cos(alpha);
R3(3,3) =  1;
end

== matlab function detumbling/DCM Kinematics/hat ==
  data: w input; w_hat output
function w_hat = hat_fcn(w)

w_hat       = zeros (3);

w_hat (1,2) = - w(3);
w_hat (1,3) =   w(2);
w_hat (2,1) =   w(3);
w_hat (2,3) = - w(1);
w_hat (3,1) = - w(2);
w_hat (3,2) =   w(1);

== matlab function detumbling/magn.vector body frame/s//c position for a given orbit/orb_elements dynamics/sat motion ==
  data: a input; orb_elements input; orb_elements_dot output
function orb_elements_dot = orbit(a,orb_elements)

mu = 3.986004418e14;

e     = orb_elements(1);
i     = orb_elements(2);
O = orb_elements(3);
o = orb_elements(4);
theta = orb_elements(5); %true anomaly


n     = sqrt( mu / a^3 ); %mean motion: angular speed required to complete 1 orbit

orb_elements_dot    = zeros (size(orb_elements));

orb_elements_dot(5) = n * (1 + e*cos(theta))^2 / (1 - e^2)^(3/2);

== matlab function detumbling/dynamic equation ==
  data: M input; u input; J input; w input; wdot output
function wdot = fcn(M,u,J,w)
%data
% J1 = 100.9e-2; %[kg m^2]
% J2 =  25.1e-2;
% J3 =  91.6e-2;
J1 = J(1);
J2 = J(2);
J3 = J(3);

% diff equation
wdot = zeros(size(w));

wdot(1) = (J2 - J3)/J1 * w(2) * w(3) + u(1)/J1 + M(1)/J1;
wdot(2) = (J3 - J1)/J2 * w(1) * w(3) + u(2)/J2 + M(2)/J2;
wdot(3) = (J1 - J2)/J3 * w(1) * w(2) + u(3)/J3 + M(3)/J3;

end

== matlab function detumbling/Disturbances: -grav.gradient -airdrag -SRP -magnetic field/SRP moment/SRP disturbance torque ==
  data: S_B input; T_srp output; A input; rho input
function T_srp = fcn(S_B,A,rho)

% Solar Radiation Pressure
F_e = 1358;
c   = 3e8;
P   =  F_e / c;

% Displaced CoM
r_CoM = 1.8e-2 * [1; 0; 0]; %considering x-axis displaced

% SC main body
n = zeros(3,10);
n(:,1) = [1; 0; 0];
n(:,2) = [0; 1; 0];
n(:,3) = [0; 0; 1];
n(:,4) = - n(:,1);
n(:,5) = - n(:,2);
n(:,6) = - n(:,3);

% % Area
% A = zeros(10,1);
% A(1) = 6*0.1*0.1; %s/c area
% A(2) = 4*0.1*0.1;
% A(3) = A(1);
% A(4) = A(1);
% A(5) = A(2);
% A(6) = A(3);
% A(7)  = 5*0.1*0.1; %solar panel area
% A(8)  = A(7);
% A(9)  = A(7);
% A(10) = A(9);

% position of center of pressure of the flat surface wrt the center of mass
r = zeros(3,10);
r(:,1) =  0.1*[1; 0; 0] - r_CoM; %typical CoP locations
r(:,2) = 0.15*[0; 1; 0] - r_CoM; %typical CoP locations
r(:,3) =  0.1*[0; 0; 1] - r_CoM; %typical CoP locations
r(:,4) = - r(:,1) - r_CoM;
r(:,5) = - r(:,2) - r_CoM;
r(:,6) = - r(:,3) - r_CoM;

rho_sMB = rho(1);
rho_dMB = rho(2);

% SC solar panels
n(:,7)  =   n(:,1);
n(:,8)  = - n(:,1);
n(:,9)  =   n(:,2);
n(:,10) = - n(:,2);

r(:,7)  =  0.25*[0; 0; 1] - r_CoM;
r(:,8)  =  r(:,7);
r(:,9)  = -0.25*[0; 0; 1] - r_CoM;
r(:,10) =  r(:,9);

rho_sSP = rho(3);
rho_dSP = rho(4);

% Forces on each side and resulting torque
F = zeros(3,10);
for i = 1:6
    if dot(S_B,n(:,i)) > 0
        F(:,i) = - P * A(i) * dot(S_B,n(:,i)) * ...
           (  (1-rho_sMB)*S_B +         ...
             ( 2*rho_sMB*dot(S_B,n(:,i)) + 2/3*rho_dMB) * n(:,i) );
    else
        F(:,i) = [0;0;0];
    end
end

for i = 7:10
    if dot(S_B,n(:,i)) > 0
        F(:,i) = - P * A(i) * dot(S_B,n(:,i)) * ...
           (  (1-rho_sSP)*S_B +         ...
             ( 2*rho_sSP*dot(S_B,n(:,i)) + 2/3*rho_dSP) * n(:,i) );
    else
        F(:,i) = [0;0;0];
    end
end

T_srp = zeros(3,1);
for i=length(F)
    T_srp = T_srp + cross(r(:,i),F(:,i));
end

end %function

== matlab function detumbling/Disturbances: -grav.gradient -airdrag -SRP -magnetic field/air drag/air drag ==
  data: vv_r input; M_drag output; A input; rho input; cd input
function M_drag = fcn(vv_r,A,rho,cd)

v_r = norm(vv_r); % 
% rho = 4.39e-16 * 1e6/1e3; %[kg/m3] rho density at constant altitude 500km
% cd = 2.2; %typical value

% Displaced CoM
r_CoM = 1.8e-2 * [1; 0; 0]; %considering x-axis displaced

% SC main body
n = zeros(3,10);
n(:,1) = [1; 0; 0];
n(:,2) = [0; 1; 0];
n(:,3) = [0; 0; 1];
n(:,4) = - n(:,1);
n(:,5) = - n(:,2);
n(:,6) = - n(:,3);
% SC solar panels
n(:,7)  =   n(:,1);
n(:,8)  = - n(:,1);
n(:,9)  =   n(:,2);
n(:,10) = - n(:,2);

% Area
% A = zeros(10,1);
% A(1) = 6*0.1*0.1;
% A(2) = 4*0.1*0.1;
% A(3) = A(1);
% A(4) = A(1);
% A(5) = A(2);
% A(6) = A(3);
% A(7)  = 5*0.1*0.1;
% A(8)  = A(7);
% A(9)  = A(7);
% A(10) = A(9);

% r: position vector from s/c CoM to CoP of surface Ai
r = zeros(3,10);
r(:,1) =  0.1*[1; 0; 0] - r_CoM; %typical CoP locations
r(:,2) = 0.15*[0; 1; 0] - r_CoM; %typical CoP locations
r(:,3) =  0.1*[0; 0; 1] - r_CoM; %typical CoP locations
r(:,4) = - r(:,1) - r_CoM;
r(:,5) = - r(:,2) - r_CoM;
r(:,6) = - r(:,3) - r_CoM;
r(:,7)  =  0.25*[0; 0; 1] - r_CoM;
r(:,8)  =  r(:,7);
r(:,9)  = -0.25*[0; 0; 1] - r_CoM;
r(:,10) =  r(:,9);

F = zeros(3,10);
M_drag = zeros(3,1);
for i=1:10
    if dot(n(:,i),vv_r/v_r) > 0
        F(:,i) = -0.5*cd*rho*v_r^2*A(i)*vv_r/v_r*dot(n(:,i),vv_r/v_r);
    end
    M_drag = M_drag + cross(r(:,i),F(:,i));
end

end %function

== matlab function detumbling/Disturbances: -grav.gradient -airdrag -SRP -magnetic field/air drag/s//c position for a given orbit/Earth's position ==
  data: a input; orb_elements input; r_N output; v_N output
function [r_N,v_N]  = Earth_pos(a,orb_elements)

mu = 3.986004418e14;

e_mod = orb_elements(1);
i     = orb_elements(2);
Omega = orb_elements(3);
omega = orb_elements(4);
theta = orb_elements(5);


h_mod = sqrt(mu*a*(1-e_mod^2));
    
e_unit = rotation_matrix_R3(-Omega) * ...
         rotation_matrix_R1(-i) * ...
         rotation_matrix_R3(-omega) * [1;0;0];
p_unit = rotation_matrix_R3(-Omega) * ...
         rotation_matrix_R1(-i) * ...
         rotation_matrix_R3(-omega) * [0;1;0];
     
r_mod_0 = h_mod^2/mu/(1+e_mod*cos(theta));
r_N       = r_mod_0 * ( cos(theta) * e_unit  +  sin(theta) * p_unit );
v_r     = mu/h_mod * e_mod*sin(theta);
v_theta = mu/h_mod * (1 + e_mod*cos(theta));
v_N       = v_r     * (  cos(theta) * e_unit  +  sin(theta) * p_unit )+ ...
          v_theta * ( -sin(theta) * e_unit  +  cos(theta) * p_unit );
end


function R1 = rotation_matrix_R1(alpha)
%{
rotation_matrix_R1: computes rotation matrix of angle alpha around x axis

INPUT:
	alpha[1]                Angle rotated
                                [rad]

OUTPUT:
    R1 [3x3]                Rotation matrix
                                [(3x3) x -]
%}

R1 = zeros(3);

R1(1,1) = 1;
R1(2,2) =  cos(alpha);
R1(2,3) =  sin(alpha);
R1(3,2) = -sin(alpha);
R1(3,3) =  cos(alpha);
end


function R3 = rotation_matrix_R3(alpha)
%{
rotation_matrix_R3: computes rotation matrix of angle alpha around z axis

INPUT:
	alpha[1]                Angle rotated
                                [rad]

OUTPUT:
    R3 [3x3]                Rotation matrix
                                [(3x3) x -]

%}

R3 = zeros(3);

R3(1,1) =  cos(alpha);
R3(1,2) =  sin(alpha);
R3(2,1) = -sin(alpha);
R3(2,2) =  cos(alpha);
R3(3,3) =  1;
end

== matlab function detumbling/Disturbances: -grav.gradient -airdrag -SRP -magnetic field/air drag/s//c position for a given orbit/orb_elements dynamics/sat motion ==
  data: a input; orb_elements input; orb_elements_dot output
function orb_elements_dot = orbit(a,orb_elements)

mu = 3.986004418e14;

e     = orb_elements(1);
i     = orb_elements(2);
O = orb_elements(3);
o = orb_elements(4);
theta = orb_elements(5); %true anomaly


n     = sqrt( mu / a^3 ); %mean motion: angular speed required to complete 1 orbit

orb_elements_dot    = zeros (size(orb_elements));

orb_elements_dot(5) = n * (1 + e*cos(theta))^2 / (1 - e^2)^(3/2);
